simulink model "test1"  (R2024b)
settings: Solver=VariableStepAuto  StartTime=0.0  StopTime=50.0  RelTol=1e-3
settings Model: Creator=francescafornasier  LastModifiedBy=yoyom
settings RTWCC: GPUComputeCapability=3.5
settings ConfigComp: CovMetricSettings=dcmwe  CovHTMLOptions=-sRT=1 -sVT=0 -aTS=1 -agT=1 -bRG=1 -bTC=1 -hTR=0 -nFC=0 -nFD=0 -scm=1 -bcm=1 -xEv=0 -xEM=0 -req=1  CovEnableCumulative=off

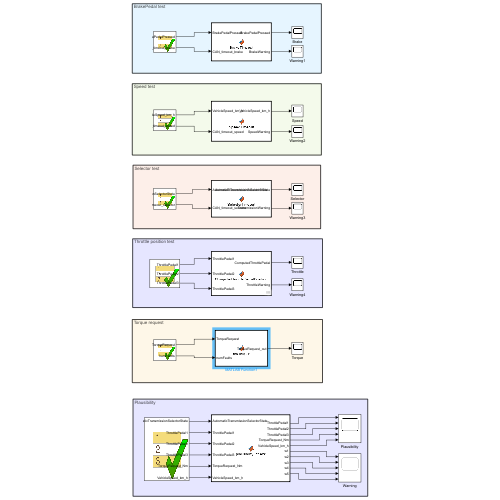
[thumbnail: Simulink's stored preview of the top-level diagram]
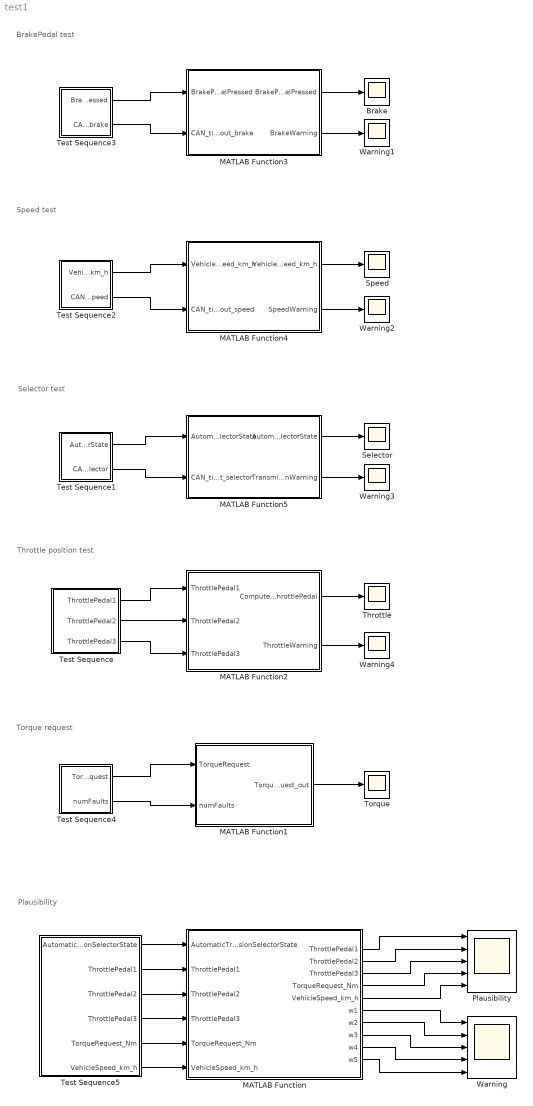
== system test1 ==
  note: Plausibility
  note: Torque request
  note: Speed test
  note: Selector test
  note: Throttle position test
  note: BrakePedal test
  Brake : Scope
  MATLAB Function : MATLAB Function  TreatAsAtomicUnit=on
  MATLAB Function1 : MATLAB Function  TreatAsAtomicUnit=on
  MATLAB Function2 : MATLAB Function  TreatAsAtomicUnit=on
  MATLAB Function3 : MATLAB Function  TreatAsAtomicUnit=on
  MATLAB Function4 : MATLAB Function  TreatAsAtomicUnit=on
  MATLAB Function5 : MATLAB Function  TreatAsAtomicUnit=on
  Plausibility : Scope  NumInputPorts=5
  Selector : Scope
  Speed : Scope
  Test Sequence : Test Sequence  TreatAsAtomicUnit=on
  Test Sequence1 : Test Sequence  TreatAsAtomicUnit=on
  Test Sequence2 : Test Sequence  TreatAsAtomicUnit=on
  Test Sequence3 : Test Sequence  TreatAsAtomicUnit=on
  Test Sequence4 : Test Sequence  TreatAsAtomicUnit=on
  Test Sequence5 : Test Sequence  TreatAsAtomicUnit=on
  Throttle : Scope
  Torque : Scope
  Warning : Scope  NumInputPorts=5
  Warning{1..4} (4 alike) : Scope
  wires:
  Test Sequence/1(ThrottlePedal1) -> MATLAB Function2/1(ThrottlePedal1)
  Test Sequence/2(ThrottlePedal2) -> MATLAB Function2/2(ThrottlePedal2)
  Test Sequence/3(ThrottlePedal3) -> MATLAB Function2/3(ThrottlePedal3)
  MATLAB Function2/2(ThrottleWarning) -> Warning4/1
  MATLAB Function5/2(TransmissionWarning) -> Warning3/1
  MATLAB Function4/2(SpeedWarning) -> Warning2/1
  MATLAB Function3/2(BrakeWarning) -> Warning1/1
  MATLAB Function2/1(ComputedThrottlePedal) -> Throttle/1
  MATLAB Function5/1(AutomaticTransmissionSelectorState) -> Selector/1
  MATLAB Function3/1(BrakePedalPressed) -> Brake/1
  MATLAB Function4/1(VehicleSpeed_km_h) -> Speed/1
  Test Sequence2/2(CAN_timeout_speed) -> MATLAB Function4/2(CAN_timeout_speed)
  Test Sequence2/1(VehicleSpeed_km_h) -> MATLAB Function4/1("VehicleSpeed_km_h ")
  Test Sequence3/2(CAN_timeout_brake) -> MATLAB Function3/2(CAN_timeout_brake)
  Test Sequence3/1(BrakePedalPressed) -> MATLAB Function3/1("BrakePedalPressed ")
  Test Sequence1/1(AutomaticTransmissionSelectorState) -> MATLAB Function5/1("AutomaticTransmissionSelectorState ")
  Test Sequence1/2(CAN_timeout_selector) -> MATLAB Function5/2(CAN_timeout_selector)
  Test Sequence4/1(TorqueRequest) -> MATLAB Function1/1(TorqueRequest)
  Test Sequence4/2(numFaults) -> MATLAB Function1/2(numFaults)
  MATLAB Function1/1(TorqueRequest_out) -> Torque/1
  Test Sequence5/2(ThrottlePedal1) -> MATLAB Function/2("ThrottlePedal1 ")
  Test Sequence5/3(ThrottlePedal2) -> MATLAB Function/3("ThrottlePedal2 ")
  Test Sequence5/4(ThrottlePedal3) -> MATLAB Function/4("ThrottlePedal3 ")
  Test Sequence5/5(TorqueRequest_Nm) -> MATLAB Function/5("TorqueRequest_Nm ")
  Test Sequence5/6(VehicleSpeed_km_h) -> MATLAB Function/6("VehicleSpeed_km_h ")
  MATLAB Function/6(w1) -> Warning/1
  MATLAB Function/7(w2) -> Warning/2
  MATLAB Function/8(w3) -> Warning/3
  MATLAB Function/9(w4) -> Warning/4
  MATLAB Function/10(w5) -> Warning/5
  MATLAB Function/5(VehicleSpeed_km_h) -> Plausibility/5
  MATLAB Function/4(TorqueRequest_Nm) -> Plausibility/4
  MATLAB Function/3(ThrottlePedal3) -> Plausibility/3
  MATLAB Function/2(ThrottlePedal2) -> Plausibility/2
  MATLAB Function/1(ThrottlePedal1) -> Plausibility/1
  Test Sequence5/1(AutomaticTransmissionSelectorState) -> MATLAB Function/1(AutomaticTransmissionSelectorState)

== stateflow chart test1/Test Sequence ==
  state step_1
    ThrottlePedal1 = single(0.5);
    ThrottlePedal2 = single(0.52);
    ThrottlePedal3 =  single(0.51);
    settings: description=All 3 signals correct
  state step_2
    ThrottlePedal1 =  single(0.55);
    ThrottlePedal2 =  single(0.52);
    ThrottlePedal3 =  single(0.5);
    settings: description=Wrong signal 1
  state step_3
    ThrottlePedal1 =  single(0.5);
    ThrottlePedal2 =  single(0.55);
    ThrottlePedal3 =  single(0.52);
    settings: description=Wrong signal 2
  state step_4
    ThrottlePedal1 =  single(0.7);
    ThrottlePedal2 =  single(0.55);
    ThrottlePedal3 =  single(0.52);
    settings: description=Wrong signal 3
  state step_5
    ThrottlePedal1 =  single(0.5);
    ThrottlePedal2 =  single(0.55);
    ThrottlePedal3 =  single(0.45);
    settings: description=All signals are different
  state step_6
    ThrottlePedal1 =  single(0.3);
    ThrottlePedal2 =  single(0.26);
    ThrottlePedal3 =  single(0.34);
    settings: description=Wrong signal 2
  (default) -> step_1
  step_1 -> step_2 : [
      | after(5, sec)
      | ]
  step_2 -> step_3 : [
      | after(5, sec)
      | ]
  step_3 -> step_4 : [
      | after(5, sec)
      | ]
  step_4 -> step_5 : [
      | after(5, sec)
      | ]
  step_5 -> step_6 : [
      | after(5, sec)
      | ]
  data: ThrottlePedal1 output; ThrottlePedal2 output; ThrottlePedal3 output

== matlab function test1/MATLAB Function3 ==
  data: BrakePedalPressed input; CAN_timeout_brake input boolean; BrakePedalPressed output; BrakeWarning output single
function [BrakePedalPressed, BrakeWarning] = BrakeTimeout(BrakePedalPressed, CAN_timeout_brake)    
    if(CAN_timeout_brake==true)
        BrakePedalPressed=true;
        BrakeWarning=single(3);
    else
        BrakeWarning=single(0);
    end

== matlab function test1/MATLAB Function4 ==
  data: VehicleSpeed_km_h input; CAN_timeout_speed input boolean; VehicleSpeed_km_h output; SpeedWarning output single
function [VehicleSpeed_km_h, SpeedWarning]= SpeedTimeout(VehicleSpeed_km_h, CAN_timeout_speed)    
    if(CAN_timeout_speed==true)
        VehicleSpeed_km_h=single(0);
        SpeedWarning=single(4);
    else
        SpeedWarning=single(0);
    end

== matlab function test1/MATLAB Function5 ==
  data: AutomaticTransmissionSelectorState output; AutomaticTransmissionSelectorState input; CAN_timeout_selector input boolean; TransmissionWarning output single
function [AutomaticTransmissionSelectorState, TransmissionWarning] = SelectorTimeout(AutomaticTransmissionSelectorState, CAN_timeout_selector)    
    if(CAN_timeout_selector==true)
        AutomaticTransmissionSelectorState=TransmissionState.Neutral;
        TransmissionWarning = single(5);
    else
        TransmissionWarning = single(0);
    end

== stateflow chart test1/Test Sequence3 ==
  state step_1
    CAN_timeout_brake = true;
    BrakePedalPressed = true;
    settings: description=Data not up to date, BrakePedalPressed = true to allow driver to chande driving mode
  state step_2
    CAN_timeout_brake = false;
    BrakePedalPressed = true;
  state step_3
    CAN_timeout_brake = false;
    BrakePedalPressed = false;
  state step_4
    CAN_timeout_brake = true;
    BrakePedalPressed = false;
  (default) -> step_1
  step_1 -> step_2 : [
      | after(5, sec)
      | ]
  step_2 -> step_3 : [
      | after(5, sec)
      | ]
  step_3 -> step_4 : [
      | after(5, sec)
      | ]
  data: BrakePedalPressed output; CAN_timeout_brake output

== matlab function test1/MATLAB Function1 ==
  data: TorqueRequest input; numFaults input; TorqueRequest_out output
function TorqueRequest_out = fcnTorque(TorqueRequest, numFaults)
    if(numFaults==2)
        TorqueRequest_out = single(0);
    else
        TorqueRequest_out = TorqueRequest;
    end

== stateflow chart test1/Test Sequence4 ==
  state step_1
    numFaults = single(0);
    TorqueRequest = single(20);
  state step_2
    numFaults = single(1);
    TorqueRequest = single(30);
  state step_3
    numFaults = single(2);
    TorqueRequest = single(25);
  (default) -> step_1
  step_1 -> step_2 : [
      | after(5, sec)
      | ]
  step_2 -> step_3 : [
      | after(5, sec)
      | ]
  data: TorqueRequest output; numFaults output

== matlab function test1/MATLAB Function ==
  data: AutomaticTransmissionSelectorState input; ThrottlePedal1 input; ThrottlePedal2 input; ThrottlePedal3 input; ThrottlePedal1 output; ThrottlePedal2 output; ThrottlePedal3 output; TorqueRequest_Nm input; TorqueRequest_Nm output; VehicleSpeed_km_h output; w1 output; w2 output; w3 output; w4 output; w5 output; VehicleSpeed_km_h input
function [ThrottlePedal1,ThrottlePedal2,ThrottlePedal3,TorqueRequest_Nm,VehicleSpeed_km_h,w1,w2,w3,w4,w5] = plausibility_check(AutomaticTransmissionSelectorState,ThrottlePedal1,ThrottlePedal2,ThrottlePedal3, TorqueRequest_Nm,VehicleSpeed_km_h)
    w1=single(0);
    w2=single(0);
    w3=single(0);
    w4=single(0);
    w5=single(0);
    if(ThrottlePedal1<0 || ThrottlePedal1>1) 
        ThrottlePedal1=single(-1);
        w1=single(1);
    end
    if(ThrottlePedal2<0 || ThrottlePedal2>1) 
        ThrottlePedal2=single(-1);
         w2=single(1);
    end
    if(ThrottlePedal3<0 || ThrottlePedal3>1) 
        ThrottlePedal3=single(-1);
         w3=single(1);
    end


    if (AutomaticTransmissionSelectorState==TransmissionState.Reverse)
        if (TorqueRequest_Nm<-40 || TorqueRequest_Nm>800)
            TorqueRequest_Nm=single(0);
            w4=single(1);
        end
    else if (TorqueRequest_Nm<-80  || TorqueRequest_Nm>80) 
        TorqueRequest_Nm=single(0);
        w4=single(2);
    end
    end



    if(VehicleSpeed_km_h<-60 || VehicleSpeed_km_h>240) 
        VehicleSpeed_km_h=single(0);
        w5=single(1);
    end

== stateflow chart test1/Test Sequence5 ==
  state step_1
    ThrottlePedal1=single(1.5);
    ThrottlePedal2=single(0.5);
    ThrottlePedal3=single(0.6);
    TorqueRequest_Nm=single(20);
    AutomaticTransmissionSelectorState=TransmissionState.Neutral;
    VehicleSpeed_km_h=single(20);
  state step_2
    ThrottlePedal1=single(-0.5);
    ThrottlePedal2=single(0.5);
    ThrottlePedal3=single(0.6);
    TorqueRequest_Nm=single(20);
    AutomaticTransmissionSelectorState=TransmissionState.Neutral;
    VehicleSpeed_km_h=single(20);
  state step_3
    ThrottlePedal1=single(0.4);
    ThrottlePedal2=single(1.2);
    ThrottlePedal3=single(0.6);
    TorqueRequest_Nm=single(20);
    AutomaticTransmissionSelectorState=TransmissionState.Neutral;
    VehicleSpeed_km_h=single(20);
  state step_4
    ThrottlePedal1=single(0.4);
    ThrottlePedal2=single(-0.3);
    ThrottlePedal3=single(0.6);
    TorqueRequest_Nm=single(20);
    AutomaticTransmissionSelectorState=TransmissionState.Neutral;
    VehicleSpeed_km_h=single(20);
  state step_5
    ThrottlePedal1=single(0.6);
    ThrottlePedal2=single(0.5);
    ThrottlePedal3=single(1.8);
    TorqueRequest_Nm=single(20);
    AutomaticTransmissionSelectorState=TransmissionState.Drive;
    VehicleSpeed_km_h=single(20);
  state step_6
    ThrottlePedal1=single(0.6);
    ThrottlePedal2=single(0.5);
    ThrottlePedal3=single(-3);
    TorqueRequest_Nm=single(20);
    AutomaticTransmissionSelectorState=TransmissionState.Neutral;
    VehicleSpeed_km_h=single(20);
  state step_7
    ThrottlePedal1=single(0.3);
    ThrottlePedal2=single(0.5);
    ThrottlePedal3=single(0.6);
    TorqueRequest_Nm=single(-70);
    AutomaticTransmissionSelectorState=TransmissionState.Reverse;
    VehicleSpeed_km_h=single(20);
  state step_8
    ThrottlePedal1=single(0.3);
    ThrottlePedal2=single(0.5);
    ThrottlePedal3=single(0.6);
    TorqueRequest_Nm=single(85);
    AutomaticTransmissionSelectorState=TransmissionState.Neutral;
    VehicleSpeed_km_h=single(20);
  state step_9
    ThrottlePedal1=single(0.3);
    ThrottlePedal2=single(0.5);
    ThrottlePedal3=single(0.6);
    TorqueRequest_Nm=single(-81);
    AutomaticTransmissionSelectorState=TransmissionState.Neutral;
    VehicleSpeed_km_h=single(20);
  state step_10
    ThrottlePedal1=single(0.3);
    ThrottlePedal2=single(0.5);
    ThrottlePedal3=single(0.6);
    TorqueRequest_Nm=single(20);
    AutomaticTransmissionSelectorState=TransmissionState.Neutral;
    VehicleSpeed_km_h=single(-100);
  state step_11
    ThrottlePedal1=single(0.3);
    ThrottlePedal2=single(0.5);
    ThrottlePedal3=single(0.6);
    TorqueRequest_Nm=single(20);
    AutomaticTransmissionSelectorState=TransmissionState.Neutral;
    VehicleSpeed_km_h=single(500);
  (default) -> step_1
  step_1 -> step_2 : [
      | after(5,sec)
      | ]
  step_2 -> step_3 : [
      | after(5,sec)
      | ]
  step_3 -> step_4 : [
      | after(5,sec)
      | ]
  step_4 -> step_5 : [
      | after(5,sec)
      | ]
  step_5 -> step_6 : [
      | after(5,sec)
      | ]
  step_6 -> step_7 : [
      | after(5,sec)
      | ]
  step_7 -> step_8 : [
      | after(5,sec)
      | ]
  step_8 -> step_9 : [
      | after(5,sec)
      | ]
  step_9 -> step_10 : [
      | after(5,sec)
      | ]
  step_10 -> step_11 : [
      | after(5,sec)
      | ]
  data: AutomaticTransmissionSelectorState output; ThrottlePedal1 output; ThrottlePedal2 output; ThrottlePedal3 output; TorqueRequest_Nm output; VehicleSpeed_km_h output

== stateflow chart test1/Test Sequence1 ==
  state step_1
    CAN_timeout_selector = false;
    AutomaticTransmissionSelectorState = TransmissionState.Drive;
  state step_2
    CAN_timeout_selector = true;
    AutomaticTransmissionSelectorState = TransmissionState.Brake;
  (default) -> step_1
  step_1 -> step_2 : [
      | after(5, sec)
      | ]
  data: AutomaticTransmissionSelectorState output Enum: TransmissionState; CAN_timeout_selector output

== matlab function test1/MATLAB Function2 ==
  data: ThrottlePedal1 input; ThrottlePedal2 input; ThrottlePedal3 input; ComputedThrottlePedal output single; ThrottleWarning output single
function [ComputedThrottlePedal,ThrottleWarning] = ComputeThrottlePedalPosition(ThrottlePedal1, ThrottlePedal2, ThrottlePedal3)
    tol = 0.05;
    ThrottleWarning=single(0);
    if(abs(ThrottlePedal1-ThrottlePedal2)<tol)
        if(abs(ThrottlePedal1-ThrottlePedal3)<tol && abs(ThrottlePedal2-ThrottlePedal3)<tol)
            ComputedThrottlePedal = mean([ThrottlePedal1 ThrottlePedal2 ThrottlePedal3]);
        else 
            ComputedThrottlePedal = mean([ThrottlePedal1 ThrottlePedal2]);
            ThrottleWarning = single(1);
        end
    elseif(abs(ThrottlePedal1-ThrottlePedal3)<tol)
            ComputedThrottlePedal = mean([ThrottlePedal1 ThrottlePedal3]);
            ThrottleWarning = single(1);
    elseif(abs(ThrottlePedal2-ThrottlePedal3)<tol)
            ComputedThrottlePedal = mean([ThrottlePedal2 ThrottlePedal3]);
            ThrottleWarning = single(1);
    else
        ThrottleWarning = single(2);
        ComputedThrottlePedal = single(-1);
    end

== stateflow chart test1/Test Sequence2 ==
  state step_1
    CAN_timeout_speed = false;
    VehicleSpeed_km_h = single(20);
  state step_2
    CAN_timeout_speed = true;
    VehicleSpeed_km_h = single(50);
  (default) -> step_1
  step_1 -> step_2 : [
      | after(5, sec)
      | ]
  data: VehicleSpeed_km_h output; CAN_timeout_speed output
